simulink library "csu_mmh_measurement_model_lib"  (R2014b)
settings: Solver=ode45  SolverMode=SingleTasking  StartTime=0.0  StopTime=10.0  RelTol=1e-3
undefined symbols (not defined in the file or in its folder): ekf_covariance_init, kfl_n_meas, kfl_state_init, kfl_target_site_planet_fixed, ldr_lander_dcm, ldr_position_in_lander
libraries: util_info_lib x1, util_quat_lib x1, util_fsw_frame_rotation_lib x1
settings Model: Creator=escrane  LastModifiedBy=escrane

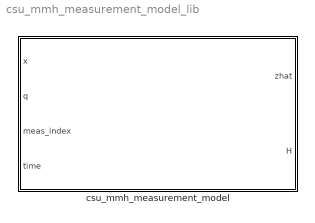
== system csu_mmh_measurement_model_lib ==
  csu_mmh_measurement_model : Subsystem

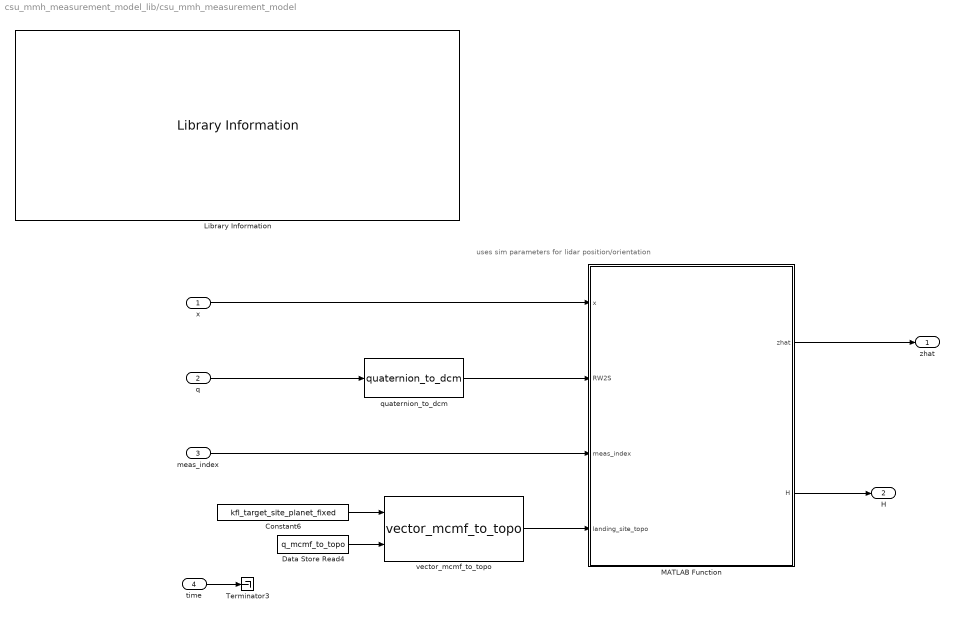
== system csu_mmh_measurement_model_lib/csu_mmh_measurement_model ==
  note: uses sim parameters for lidar position/orientation
  x : Inport
  q : Inport  Port=2
  meas_index : Inport  Port=3
  time : Inport  Port=4
  Constant6 : Constant  Value=kfl_target_site_planet_fixed  VectorParams1D=off
  Data Store Read4 : DataStoreRead  DataStoreName=q_mcmf_to_topo
  Library Information : util_info_lib/Library Information  owner='NONE'
  MATLAB Function : MATLAB Function  TreatAsAtomicUnit=on
  Terminator3 : Terminator
  quaternion_to_dcm : util_quat_lib/quaternion_to_dcm  SystemSampleTime=-1
  vector_mcmf_to_topo : util_fsw_frame_rotation_lib/vector_mcmf_to_topo  SystemSampleTime=-1
  zhat : Outport  InitialOutput=kfl_state_init
  H : Outport  Port=2  InitialOutput=ekf_covariance_init
  wires:
  Data Store Read4/1 -> vector_mcmf_to_topo/2
  time/1 -> Terminator3/1
  vector_mcmf_to_topo/1 -> MATLAB Function/4(landing_site_topo)
  Constant6/1 -> vector_mcmf_to_topo/1
  q/1 -> quaternion_to_dcm/1
  quaternion_to_dcm/1 -> MATLAB Function/2(RW2S)
  x/1 -> MATLAB Function/1(x)
  MATLAB Function/1(zhat) -> zhat/1
  MATLAB Function/2(H) -> H/1
  meas_index/1 -> MATLAB Function/3(meas_index)

== matlab function csu_mmh_measurement_model_lib/csu_mmh_measurement_model/MATLAB Function ==
  data: x input size=[kfl_n_state 1]; zhat output double size=[kfl_n_meas 1]; RW2S input size=[3 3]; H output size=[kfl_n_meas kfl_n_state]; meas_index input size=[kfl_n_meas 1]; kfl_n_meas parameter; landing_site_topo input; ldr_position_in_lander parameter; ldr_lander_dcm parameter
function [zhat, H] = construct_measurement_model(x, RW2S, meas_index, kfl_n_meas, landing_site_topo, ldr_position_in_lander, ldr_lander_dcm)
%#codegen

H = zeros(6,15);
zhat = zeros(6,1);
  

%---------------------------------------------------------------------s%
% lidar
T = x(1:3) + ( RW2S * ldr_position_in_lander' ) ; 
RW2C = ldr_lander_dcm *  RW2S ;

ground_normal_topo = [0 0 1]';


for ii = 1 : kfl_n_meas
    
    switch meas_index(ii)
        
        case 1
            % slant range update
            u = [0 0 1]'; % nadir pointing radar
            
            radar_denominator =  ground_normal_topo'*(RW2C'*u);
            range_hat = (ground_normal_topo' * (-T)) / radar_denominator;
            zhat(ii) = range_hat;
            
            
            H(1, 1) = -ground_normal_topo(1) / radar_denominator;

            H(1, 2) = -ground_normal_topo(2) / radar_denominator;

            H(1, 3) = -ground_normal_topo(3) / radar_denominator;
            
        % homography velocity measurement
        % Model is element 4 of state vector, x velocity
        case 2
            H(meas_index(ii), 4) = 1;
            zhat(ii) = x(4);
            
        % homography velocity measurement
        % Model is element 5 of state vector, y velocity
        case 3
            H(meas_index(ii), 5) = 1;
            zhat(ii) = x(5);
            
        % star tracker: direct gibbs vector measurement (frames already taken care of)
        % Model is element 10 of state vector
        case 4
            H(meas_index(ii), 10) = 1;
            zhat(ii) = x(10);
            
        % Model is element 11 of state vector
        case 5
            H(meas_index(ii), 11) = 1;
            zhat(ii) = x(11);
            
         % Model is element 12 of state vector
        case 6
            H(meas_index(ii), 12) = 1;
            zhat(ii) = x(12);
          
        otherwise
            % no update: no valid measurement in this slot
            
    end
    
end
